simulink model "ITCG_3D_FOV_simulation"  (R2023b)
settings: Solver=FixedStepAuto  StartTime=0.0  StopTime=t_d  FixedStep=1/100  RelTol=1e-3
values from neighbouring files (symbols this model uses):
  K = 8    [ITCG_FOV_plot.m]    (also in ITCG_FOV_plot_one.m; ITCG_FOV_sim.m = j)
  N = 3    [ITCG_FOV_plot.m]    (also in ITCG_FOV_plot_one.m = N_range(i); ITCG_FOV_sim.m = i)
  n = 5    [ITCG_FOV_plot.m]    (also in ITCG_FOV_plot_one.m; ITCG_FOV_sim.m = g)
  sigma_max = sigma_max_range(i)    [ITCG_FOV_plot.m]    (also in ITCG_FOV_plot_one.m = 45; ITCG_FOV_sim.m = s)
  t_d = 23    [ITCG_FOV_plot.m]    (also in ITCG_FOV_plot_one.m = 30; ITCG_FOV_sim.m = l)
libraries: simulink_extras x2, simulink x1
settings Model: NumberOfSteps=10  PacingRate=5  Creator=Administrator  LastModifiedBy=lmj04
settings DebuggingCC: UnderSpecifiedDimensionMsg=warning

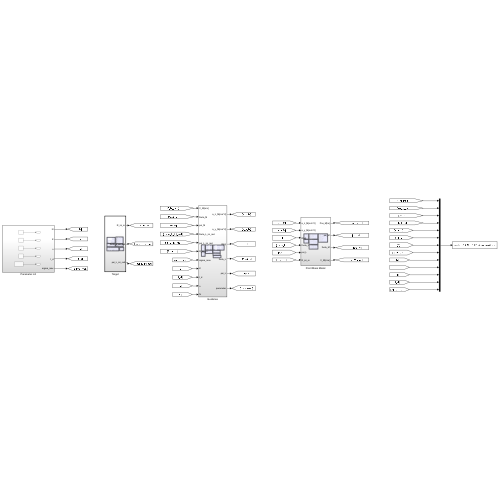
[thumbnail: Simulink's stored preview of the top-level diagram]
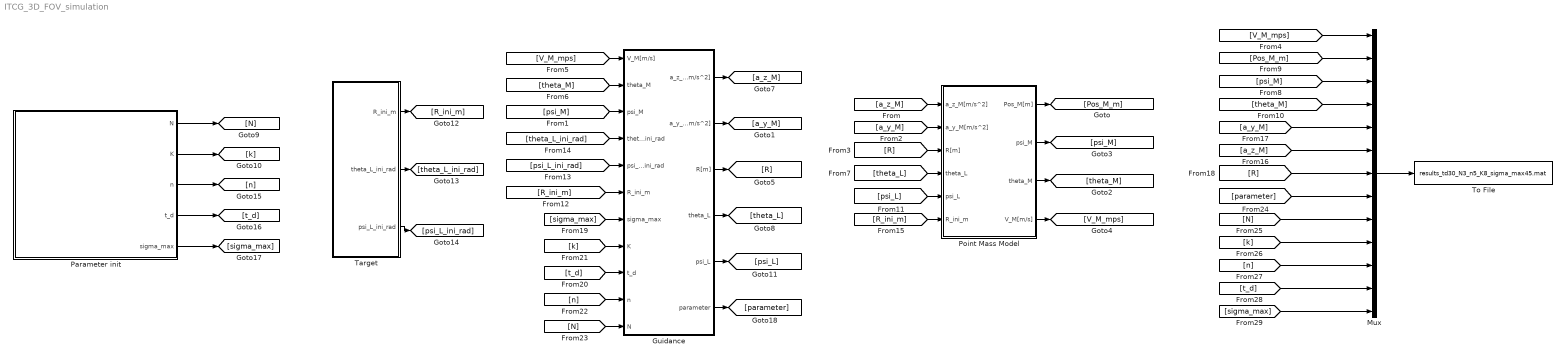
== system ITCG_3D_FOV_simulation ==
  Guidance : Subsystem
  Mux : Mux  Inputs=13
  Parameter init : Subsystem
  Point Mass Model : Subsystem
  Target : Subsystem  TreatAsAtomicUnit=on
  To File : ToFile  Filename=results_td30_N3_n5_K8_sigma_max45.mat
  wires:
  [V_M_mps] -> Guidance/1(V_M[m/s])
  [theta_M] -> Guidance/2(theta_M)
  [psi_M] -> Guidance/3(psi_M)
  Target/1(R_ini_m) -> [R_ini_m]
  Target/2(theta_L_ini_rad) -> [theta_L_ini_rad]
  Target/3(psi_L_ini_rad) -> [psi_L_ini_rad]
  Guidance/5(psi_L) -> [psi_L]
  Guidance/1(a_z_M[m/s^2]) -> [a_z_M]
  Guidance/2(a_y_M[m/s^2]) -> [a_y_M]
  Guidance/3(R[m]) -> [R]
  Guidance/4(theta_L) -> [theta_L]
  [a_z_M] -> Point Mass Model/1(a_z_M[m/s^2])
  [a_y_M] -> Point Mass Model/2(a_y_M[m/s^2])
  [R] -> Point Mass Model/3(R[m])
  [theta_L] -> Point Mass Model/4(theta_L)
  [psi_L] -> Point Mass Model/5(psi_L)
  Point Mass Model/1(Pos_M[m]) -> [Pos_M_m]
  Point Mass Model/2(psi_M) -> [psi_M]
  Point Mass Model/3(theta_M) -> [theta_M]
  Point Mass Model/4(V_M[m/s]) -> [V_M_mps]
  [R_ini_m] -> Guidance/6(R_ini_m)
  [psi_L_ini_rad] -> Guidance/5(psi_L_ini_rad)
  [theta_L_ini_rad] -> Guidance/4(theta_L_ini_rad)
  [R_ini_m] -> Point Mass Model/6(R_ini_m)
  Parameter init/4(t_d) -> [t_d]
  Parameter init/1(N) -> [N]
  Parameter init/3(n) -> [n]
  Parameter init/2(K) -> [k]
  Parameter init/5(sigma_max) -> [sigma_max]
  [sigma_max] -> Guidance/7(sigma_max)
  [t_d] -> Guidance/9(t_d)
  [k] -> Guidance/8(K)
  [n] -> Guidance/10(n)
  [N] -> Guidance/11(N)
  Guidance/6(parameter) -> [parameter]
  [V_M_mps] -> Mux/1
  [Pos_M_m] -> Mux/2
  [psi_M] -> Mux/3
  [theta_M] -> Mux/4
  [a_y_M] -> Mux/5
  [a_z_M] -> Mux/6
  [R] -> Mux/7
  [parameter] -> Mux/8
  [N] -> Mux/9
  [k] -> Mux/10
  [n] -> Mux/11
  [t_d] -> Mux/12
  [sigma_max] -> Mux/13
  Mux/1 -> To File/1

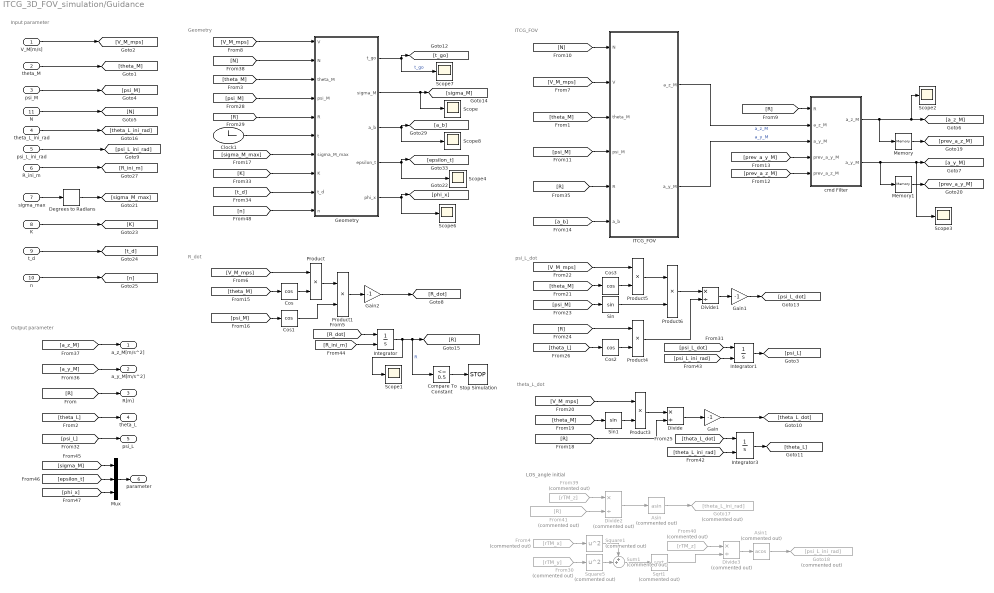
== system ITCG_3D_FOV_simulation/Guidance ==
  note: Input parameter
  note: ITCG_FOV
  note: R_dot
  note: psi_L_dot
  note: theta_L_dot
  note: Geometry
  note: Output parameter
  note: LOS_angle initial
  V_M[m/s] : Inport
  theta_M : Inport  Port=2
  psi_M : Inport  Port=3
  theta_L_ini_rad : Inport  Port=4
  psi_L_ini_rad : Inport  Port=5
  R_ini_m : Inport  Port=6
  sigma_max : Inport  Port=7
  K : Inport  Port=8
  t_d : Inport  Port=9
  n : Inport  Port=10
  N : Inport  Port=11
  Asin : Trigonometry  Commented=on  Operator=asin
  Asin1 : Trigonometry  Commented=on  Operator=acos
  Clock1 : Clock
  Compare To Constant : simulink/Logic and Bit Operations/Compare To Constant  relop=<=  const=0.5  OutDataTypeStr=boolean
  Cos{,1..3} (4 alike) : Trigonometry  Operator=cos
  Degrees to Radians : simulink_extras/Transformations/Degrees to Radians
  Divide : Product  Inputs=*/
  Divide1 : Product  Inputs=*/
  Divide2 : Product  Commented=on  Inputs=*/
  Divide3 : Product  Commented=on  Inputs=*/
  From30 : From  Commented=on  GotoTag=rTM_y
  From39 : From  Commented=on  GotoTag=rTM_z
  From4 : From  Commented=on  GotoTag=rTM_x
  From40 : From  Commented=on  GotoTag=rTM_z
  From41 : From  Commented=on  GotoTag=R
  Gain : Gain  Gain=-1
  Gain1 : Gain  Gain=-1
  Gain2 : Gain  Gain=-1
  Geometry : MATLAB Function  TreatAsAtomicUnit=on
  Goto17 : Goto  Commented=on  GotoTag=theta_L_ini_rad
  Goto18 : Goto  Commented=on  GotoTag=psi_L_ini_rad
  ITCG_FOV : MATLAB Function  TreatAsAtomicUnit=on
  Integrator : Integrator  InitialConditionSource=external  InitialCondition=sqrt(300^2+500^2+200^2)
  Integrator1 : Integrator  InitialConditionSource=external
  Integrator3 : Integrator  InitialConditionSource=external
  Memory : Memory
  Memory1 : Memory
  Mux : Mux  Inputs=3
  Product{,1,3..6} (6 alike) : Product
  Scope{,1..4,6..8} (8 alike) : Scope
  Sin : Trigonometry
  Sin1 : Trigonometry
  Sqrt1 : Sqrt  Commented=on
  Square1 : Math  Commented=on  Operator=square
  Square5 : Math  Commented=on  Operator=square
  Stop Simulation : Stop
  Sum1 : Sum  Commented=on  Inputs=++|
  cmd Filter : MATLAB Function  TreatAsAtomicUnit=on
  a_z_M[m/s^2] : Outport
  a_y_M[m/s^2] : Outport  Port=2
  R[m] : Outport  Port=3
  theta_L : Outport  Port=4
  psi_L : Outport  Port=5
  parameter : Outport  Port=6
  wires:
  V_M[m/s]/1 -> [V_M_mps]
  N/1 -> [N]
  theta_M/1 -> [theta_M]
  psi_M/1 -> [psi_M]
  Product1/1 -> Gain2/1
  [R] -> Geometry/5(R)
  Gain2/1 -> [R_dot]
  [theta_L] -> Cos2/1
  [theta_L_dot] -> Integrator3/1
  [theta_M] -> Geometry/3(theta_M)
  Gain/1 -> [theta_L_dot]
  Product5/1 -> Product6/1
  Divide1/1 -> Gain1/1
  [V_M_mps] -> Product3/1
  [V_M_mps] -> Geometry/1(V)
  [psi_M] -> Geometry/4(psi_M)
  [V_M_mps] -> Product5/1
  [theta_M] -> Sin1/1
  [R] -> Divide/2
  [theta_M] -> Cos3/1
  [psi_M] -> ITCG_FOV/4(psi_M)
  Divide/1 -> Gain/1
  [theta_M] -> Cos/1
  [R] -> Product4/1
  Product4/1 -> Divide1/2
  Integrator3/1 -> [theta_L]
  [psi_L_dot] -> Integrator1/1
  Sin1/1 -> Product3/2
  Product3/1 -> Divide/1
  [psi_M] -> Cos1/1
  Cos/1 -> Product/2
  Integrator1/1 -> [psi_L]
  [N] -> ITCG_FOV/1(N)
  [theta_M] -> ITCG_FOV/3(theta_M)
  Product6/1 -> Divide1/1
  [psi_M] -> Sin/1
  Compare To Constant/1 -> Stop Simulation/1
  [V_M_mps] -> Product/1
  Cos3/1 -> Product5/2
  Sin/1 -> Product6/2
  Integrator/1 -> Scope1/1, [R], Compare To Constant/1  "R"
  [R] -> ITCG_FOV/5(R)
  Product/1 -> Product1/1
  Geometry/1(t_go) -> [t_go], Scope7/1  "t_go"
  Cos2/1 -> Product4/2
  Cos1/1 -> Product1/2
  Gain1/1 -> [psi_L_dot]
  [R_dot] -> Integrator/1
  [V_M_mps] -> ITCG_FOV/2(V)
  [N] -> Geometry/2(N)
  [a_z_M] -> a_z_M[m/s^2]/1
  [theta_L] -> theta_L/1
  [psi_L] -> psi_L/1
  [R] -> R[m]/1
  [a_y_M] -> a_y_M[m/s^2]/1
  [psi_L_ini_rad] -> Integrator1/2
  [theta_L_ini_rad] -> Integrator3/2
  [R_ini_m] -> Integrator/2
  R_ini_m/1 -> [R_ini_m]
  Divide3/1 -> Asin1/1
  Sum1/1 -> Sqrt1/1
  From30/1 -> Square5/1
  Square5/1 -> Sum1/2
  Square1/1 -> Sum1/1
  Asin/1 -> Goto17/1
  Sqrt1/1 -> Divide3/2
  From41/1 -> Divide2/2
  Asin1/1 -> Goto18/1
  From40/1 -> Divide3/1
  From39/1 -> Divide2/1
  From4/1 -> Square1/1
  Divide2/1 -> Asin/1
  theta_L_ini_rad/1 -> [theta_L_ini_rad]
  psi_L_ini_rad/1 -> [psi_L_ini_rad]
  Clock1/1 -> Geometry/6(t)
  Geometry/3(a_b) -> [a_b], Scope8/1
  Geometry/4(epsilon_t) -> [epsilon_t], Scope4/1
  [a_b] -> ITCG_FOV/6(a_b)
  sigma_max/1 -> Degrees to Radians/1
  Degrees to Radians/1 -> [sigma_M_max]
  [sigma_M_max] -> Geometry/7(sigma_M_max)
  Geometry/5(phi_x) -> [phi_x], Scope6/1
  K/1 -> [K]
  t_d/1 -> [t_d]
  [K] -> Geometry/8(K)
  [t_d] -> Geometry/9(t_d)
  ITCG_FOV/1(a_z_M) -> cmd Filter/2("a_z_M ")  "a_z_M"
  ITCG_FOV/2(a_y_M) -> cmd Filter/3("a_y_M ")  "a_y_M"
  [R] -> cmd Filter/1(R)
  cmd Filter/1(a_z_M) -> Memory/1, Scope2/1, [a_z_M]
  cmd Filter/2(a_y_M) -> Scope3/1, [a_y_M], Memory1/1
  Memory/1 -> [prev_a_z_M]
  Memory1/1 -> [prev_a_y_M]
  [prev_a_z_M] -> cmd Filter/5(prev_a_z_M)
  [prev_a_y_M] -> cmd Filter/4(prev_a_y_M)
  n/1 -> [n]
  [n] -> Geometry/10(n)
  [sigma_M] -> Mux/1
  [epsilon_t] -> Mux/2
  [phi_x] -> Mux/3
  Mux/1 -> parameter/1
  Geometry/2(sigma_M) -> [sigma_M], Scope/1

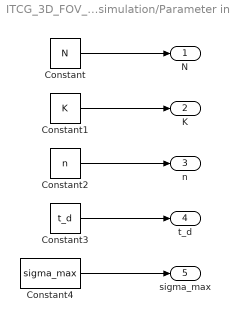
== system ITCG_3D_FOV_simulation/Parameter init ==
  Constant : Constant  Value=N
  Constant1 : Constant  Value=K
  Constant2 : Constant  Value=n
  Constant3 : Constant  Value=t_d
  Constant4 : Constant  Value=sigma_max
  N : Outport
  K : Outport  Port=2
  n : Outport  Port=3
  t_d : Outport  Port=4
  sigma_max : Outport  Port=5
  wires:
  Constant/1 -> N/1
  Constant1/1 -> K/1
  Constant2/1 -> n/1
  Constant3/1 -> t_d/1
  Constant4/1 -> sigma_max/1

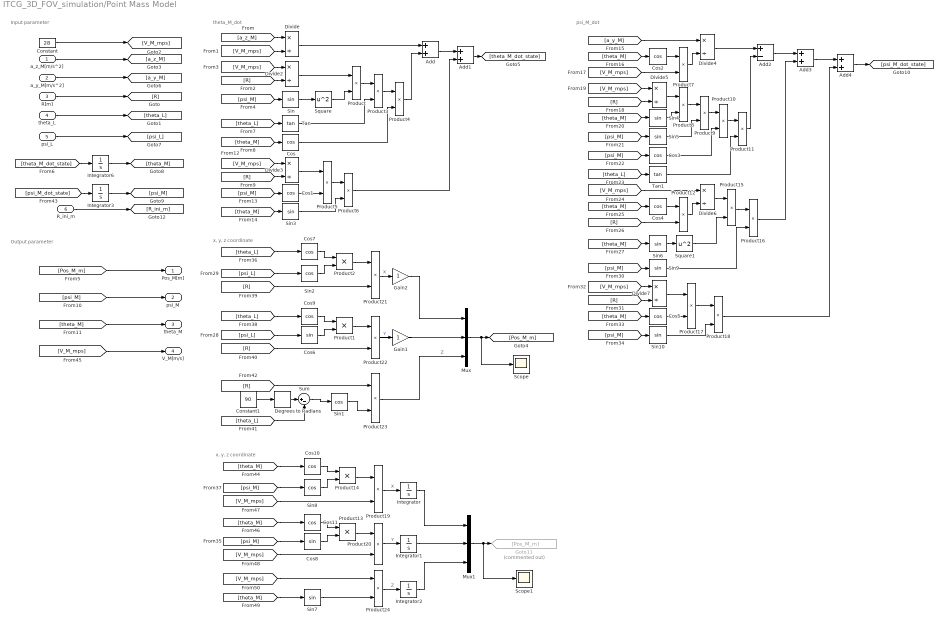
== system ITCG_3D_FOV_simulation/Point Mass Model ==
  note: Input parameter
  note: x, y, z coordinate
  note: theta_M_dot
  note: Output parameter
  note: psi_M_dot
  note: x, y, z coordinate
  a_z_M[m/s^2] : Inport
  a_y_M[m/s^2] : Inport  Port=2
  R[m] : Inport  Port=3
  theta_L : Inport  Port=4
  psi_L : Inport  Port=5
  R_ini_m : Inport  Port=6
  Add{,1,3..4} (4 alike) : Sum
  Add2 : Sum  Inputs=+-
  Constant : Constant  Value=28
  Constant1 : Constant  Value=90
  Cos{,1..5,7,9..11} (10 alike) : Trigonometry  Operator=cos
  Cos6 : Trigonometry
  Cos8 : Trigonometry
  Degrees to Radians : simulink_extras/Transformations/Degrees to Radians
  Divide{,2..7} (7 alike) : Product  Inputs=*/
  Gain1 : Gain
  Gain2 : Gain
  Goto11 : Goto  Commented=on  GotoTag=Pos_M_m
  Integrator : Integrator
  Integrator1 : Integrator
  Integrator2 : Integrator
  Integrator3 : Integrator  InitialCondition=10*pi/180
  Integrator6 : Integrator  InitialCondition=10*pi/180
  Mux : Mux  Inputs=3
  Mux1 : Mux  Inputs=3
  Product{,1..24} (25 alike) : Product
  Scope : Scope
  Scope1 : Scope
  Sin{,3..7,9..10} (8 alike) : Trigonometry
  Sin1 : Trigonometry  Operator=cos
  Sin2 : Trigonometry  Operator=cos
  Sin8 : Trigonometry  Operator=cos
  Square : Math  Operator=square
  Square1 : Math  Operator=square
  Sum : Sum  Inputs=|+-
  Tan : Trigonometry  Operator=tan
  Tan1 : Trigonometry  Operator=tan
  Pos_M[m] : Outport
  psi_M : Outport  Port=2
  theta_M : Outport  Port=3
  V_M[m/s] : Outport  Port=4
  wires:
  [theta_L] -> Tan1/1
  Product16/1 -> Add3/2
  Product9/1 -> Product10/1
  [psi_M] -> psi_M/1
  Tan/1 -> Product3/2
  [psi_M_dot_state] -> Integrator3/1
  [psi_M] -> Sin9/1
  [theta_M] -> Cos/1
  Sin10/1 -> Product18/2
  [psi_M] -> Sin5/1
  Product17/1 -> Product18/1
  [psi_M] -> Sin10/1
  [theta_L] -> Cos9/1
  [V_M_mps] -> Divide/2
  Sin6/1 -> Square1/1
  Product15/1 -> Product16/1
  [V_M_mps] -> V_M[m/s]/1
  Cos5/1 -> Product17/2
  Sin/1 -> Square/1
  Add2/1 -> Add3/1
  Divide7/1 -> Product17/1
  [theta_M] -> Sin6/1
  [R] -> Divide7/2
  Sin3/1 -> Product6/2
  Add1/1 -> [theta_M_dot_state]
  Sin9/1 -> Product16/2
  Divide6/1 -> Product15/1
  Square1/1 -> Product15/2
  [R] -> Divide3/2
  [a_z_M] -> Divide/1
  [theta_M] -> Cos5/1
  Add3/1 -> Add4/1
  Product12/1 -> Divide6/2
  Product8/1 -> Product9/1
  [a_y_M] -> Divide4/1
  [psi_M] -> Cos3/1
  Product10/1 -> Product11/1
  Product3/1 -> Product4/1
  Divide4/1 -> Add2/1
  Cos3/1 -> Product10/2
  Product11/1 -> Add2/2
  [R] -> Product12/2
  [V_M_mps] -> Divide5/1
  Cos/1 -> Product4/2
  Product5/1 -> Product6/1
  Product6/1 -> Add1/2
  Divide3/1 -> Product5/1
  Cos1/1 -> Product5/2
  Square/1 -> Product/2
  theta_L/1 -> [theta_L]
  [psi_M] -> Cos1/1
  [V_M_mps] -> Product7/2
  [R] -> Divide2/2
  Cos6/1 -> Product1/2
  [V_M_mps] -> Divide2/1
  [psi_M] -> Sin/1
  a_y_M[m/s^2]/1 -> [a_y_M]
  [theta_M] -> Sin4/1
  Tan1/1 -> Product11/2
  Product23/1 -> Mux/3  "Z"
  [Pos_M_m] -> Pos_M[m]/1
  Integrator6/1 -> [theta_M]
  [theta_M] -> Sin3/1
  [psi_L] -> Cos6/1
  Add/1 -> Add1/1
  psi_L/1 -> [psi_L]
  [R] -> Divide5/2
  Product21/1 -> Gain2/1  "X"
  [V_M_mps] -> Divide6/1
  Product1/1 -> Product22/1
  Integrator3/1 -> [psi_M]
  Product/1 -> Product3/1
  Sin2/1 -> Product2/2
  a_z_M[m/s^2]/1 -> [a_z_M]
  Add4/1 -> [psi_M_dot_state]
  [V_M_mps] -> Divide7/1
  Cos2/1 -> Product7/1
  Mux/1 -> [Pos_M_m], Scope/1
  R[m]/1 -> [R]
  [theta_M] -> theta_M/1
  [psi_L] -> Sin2/1
  Constant/1 -> [V_M_mps]
  Divide2/1 -> Product/1
  [theta_M] -> Cos2/1
  Sin4/1 -> Product8/2
  [theta_L] -> Tan/1
  Cos4/1 -> Product12/1
  Product2/1 -> Product21/1
  [theta_M] -> Cos4/1
  Cos9/1 -> Product1/1
  [V_M_mps] -> Divide3/1
  Sin5/1 -> Product9/2
  [theta_L] -> Cos7/1
  Product4/1 -> Add/2
  Product18/1 -> Add4/2
  Product7/1 -> Divide4/2
  Divide5/1 -> Product8/1
  Divide/1 -> Add/1
  Cos7/1 -> Product2/1
  [theta_M_dot_state] -> Integrator6/1
  Product22/1 -> Gain1/1  "Y"
  [V_M_mps] -> Product24/1
  Sin7/1 -> Product24/2
  [V_M_mps] -> Product20/2
  [theta_M] -> Cos11/1
  [psi_M] -> Sin8/1
  Mux1/1 -> Scope1/1, Goto11/1
  [theta_M] -> Sin7/1
  Sin8/1 -> Product14/2
  Product14/1 -> Product19/1
  Product19/1 -> Integrator/1  "X"
  Product13/1 -> Product20/1
  Product24/1 -> Integrator2/1  "Z"
  [psi_M] -> Cos8/1
  [V_M_mps] -> Product19/2
  [theta_M] -> Cos10/1
  Cos11/1 -> Product13/1
  Cos8/1 -> Product13/2
  Product20/1 -> Integrator1/1  "Y"
  Cos10/1 -> Product14/1
  Integrator/1 -> Mux1/1
  Integrator1/1 -> Mux1/2
  Integrator2/1 -> Mux1/3
  R_ini_m/1 -> [R_ini_m]
  [R] -> Product21/2
  [R] -> Product22/2
  Gain1/1 -> Mux/2
  Gain2/1 -> Mux/1
  [R] -> Product23/1
  Constant1/1 -> Degrees to Radians/1
  Degrees to Radians/1 -> Sum/1
  Sin1/1 -> Product23/2
  [theta_L] -> Sum/2
  Sum/1 -> Sin1/1

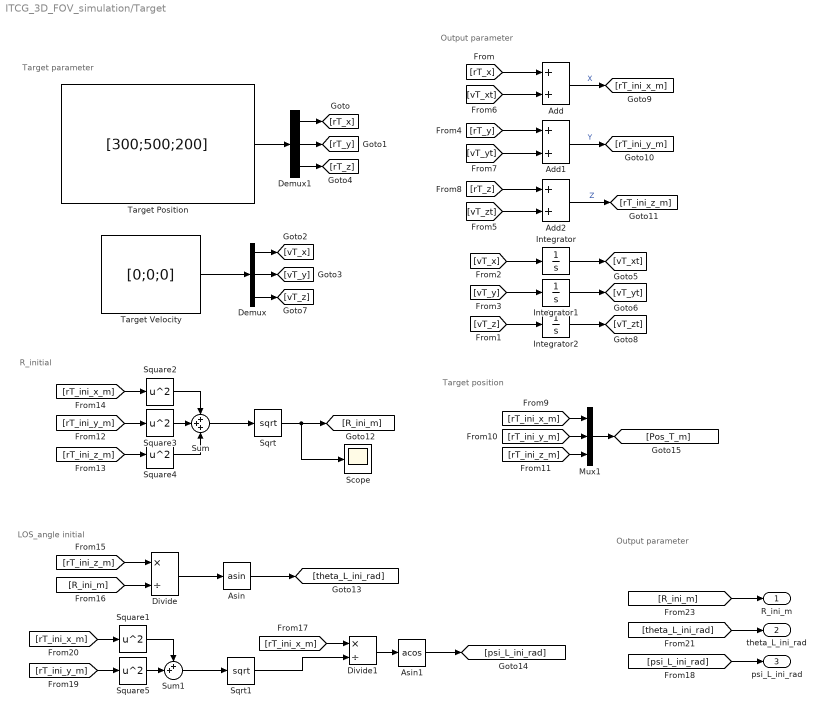
== system ITCG_3D_FOV_simulation/Target ==
  note: LOS_angle initial
  note: Target position
  note: Target parameter
  note: Output parameter
  note: R_initial
  note: Output parameter
  Add : Sum
  Add1 : Sum
  Add2 : Sum
  Asin : Trigonometry  Operator=asin
  Asin1 : Trigonometry  Operator=acos
  Demux : Demux  Outputs=3
  Demux1 : Demux  Outputs=3
  Divide : Product  Inputs=*/
  Divide1 : Product  Inputs=*/
  Integrator : Integrator
  Integrator1 : Integrator
  Integrator2 : Integrator
  Mux1 : Mux  Inputs=3
  Scope : Scope
  Sqrt : Sqrt
  Sqrt1 : Sqrt
  Square{1..5} (5 alike) : Math  Operator=square
  Sum : Sum  Inputs=+++
  Sum1 : Sum  Inputs=++|
  Target Position : Constant  Value=[300;500;200]  VectorParams1D=off
  Target Velocity : Constant  Value=[0;0;0]  VectorParams1D=off
  R_ini_m : Outport
  theta_L_ini_rad : Outport  Port=2
  psi_L_ini_rad : Outport  Port=3
  wires:
  [psi_L_ini_rad] -> psi_L_ini_rad/1
  Asin/1 -> [theta_L_ini_rad]
  [rT_ini_z_m] -> Mux1/3
  [rT_z] -> Add2/1
  Demux/3 -> [vT_z]
  [vT_z] -> Integrator2/1
  Demux/2 -> [vT_y]
  [rT_ini_x_m] -> Mux1/1
  Add1/1 -> [rT_ini_y_m]  "Y"
  Square2/1 -> Sum/1
  [vT_x] -> Integrator/1
  Mux1/1 -> [Pos_T_m]
  Square3/1 -> Sum/2
  Add2/1 -> [rT_ini_z_m]  "Z"
  Target Position/1 -> Demux1/1
  Integrator/1 -> [vT_xt]
  Sum/1 -> Sqrt/1
  Demux1/3 -> [rT_z]
  [rT_ini_y_m] -> Mux1/2
  Integrator1/1 -> [vT_yt]
  Demux/1 -> [vT_x]
  Demux1/1 -> [rT_x]
  Target Velocity/1 -> Demux/1
  Demux1/2 -> [rT_y]
  Add/1 -> [rT_ini_x_m]  "X"
  [vT_yt] -> Add1/2
  Divide1/1 -> Asin1/1
  [rT_x] -> Add/1
  [vT_zt] -> Add2/2
  Sum1/1 -> Sqrt1/1
  [rT_ini_x_m] -> Square1/1
  Square1/1 -> Sum1/1
  Square5/1 -> Sum1/2
  [rT_ini_y_m] -> Square5/1
  [vT_y] -> Integrator1/1
  [rT_y] -> Add1/1
  [rT_ini_x_m] -> Square2/1
  [rT_ini_z_m] -> Divide/1
  [R_ini_m] -> R_ini_m/1
  Sqrt/1 -> Scope/1, [R_ini_m]
  [R_ini_m] -> Divide/2
  [rT_ini_z_m] -> Square4/1
  [rT_ini_y_m] -> Square3/1
  Sqrt1/1 -> Divide1/2
  [vT_xt] -> Add/2
  Divide/1 -> Asin/1
  Integrator2/1 -> [vT_zt]
  Square4/1 -> Sum/3
  [rT_ini_x_m] -> Divide1/1
  [theta_L_ini_rad] -> theta_L_ini_rad/1
  Asin1/1 -> [psi_L_ini_rad]

== matlab function ITCG_3D_FOV_simulation/Guidance/Geometry ==
  data: V input; N input; t_go output; sigma_M output; theta_M input; psi_M input; R input; t input; a_b output; epsilon_t output; sigma_M_max input; phi_x output; K input; t_d input; n input
function [t_go, sigma_M, a_b, epsilon_t, phi_x] =fcn(V, N, theta_M, psi_M, R, t, sigma_M_max, K, t_d, n)
    D2R=pi/180;
    sigma_M=acos(cos(theta_M)*cos(psi_M));
    t_go = (R / V) * (1 + (sigma_M^2 / ( 2 * (2 * N - 1) ) ) );
    epsilon_t = t_d-t_go-t;
    x = sigma_M/sigma_M_max;
    
    phi_x = 1-abs(x)^n;
    % phi_x = (1/(1-exp(-1))) * (exp(-abs(x)^n)-exp(-1));
    % phi_x = cos(pi*x^n/2);

    t_go = (R / V) * (1 + (sigma_M^2 / ( 2 * (2 * N - 1) ) ) );
    a_b = ((K*phi_x*(2*N-1)*V^2) / (R*t_go*sin(sigma_M)^2))*epsilon_t ;

== matlab function ITCG_3D_FOV_simulation/Guidance/cmd Filter ==
  data: R input; a_z_M output; a_z_M input; a_y_M input; prev_a_y_M input; prev_a_z_M input; a_y_M output
function [a_z_M, a_y_M] = fcn(R, a_z_M, a_y_M, prev_a_y_M, prev_a_z_M)

if R<10
    a_z_M = prev_a_z_M;
    a_y_M = prev_a_y_M;
end

== matlab function ITCG_3D_FOV_simulation/Guidance/ITCG_FOV ==
  data: a_z_M output; a_y_M output; N input; V input; theta_M input; psi_M input; R input; a_b input
function [a_z_M, a_y_M]  = fcn(N, V, theta_M, psi_M, R, a_b)
   
    a_y_PNG = -N*V^2/R*sin(psi_M);
    a_z_PNG = -N*V^2/R*sin(theta_M)*cos(psi_M);
    % e_a = [0, sin(psi)/sin(sigma_M), sin(theta_M)*cos(psi)/sin(sigma_M)];

    %% ITCG_FOV command

    % a_y_M = ((-N*V^2/R)*sin(sigma_M)+(K*phi_x*(2*N-1)*V^2)/(R*t_go*sin(sigma_M))*epsilon_t) * (sin(psi_M)/sin(sigma_M));
    % a_z_M = ((-N*V^2/R)*sin(sigma_M)+(K*phi_x*(2*N-1)*V^2)/(R*t_go*sin(sigma_M))*epsilon_t) * (sin(theta_M)*cos(psi_M)/sin(sigma_M));

    a_y_M = a_y_PNG + a_b*sin(psi_M);
    a_z_M = a_z_PNG + a_b*sin(theta_M)*cos(psi_M);
